simulink model "create_desRN_Test"  (R2024b)
settings: Solver=VariableStepAuto  StartTime=0.0  StopTime=10.0  RelTol=1e-3
settings Model: Creator=AdamY  LastModifiedBy=AdamY

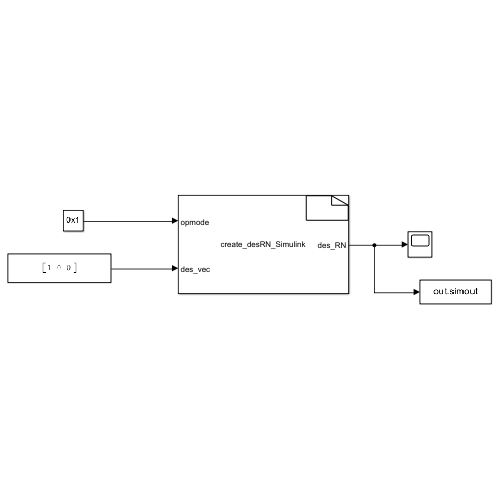
[thumbnail: Simulink's stored preview of the top-level diagram]
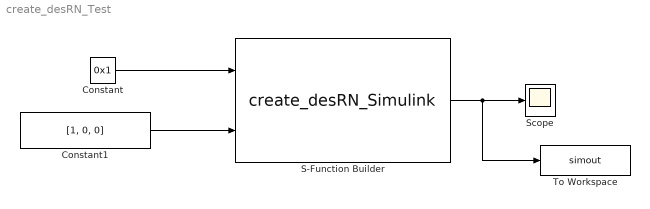
== system create_desRN_Test ==
  Constant : Constant  Value=0x1  OutDataTypeStr=uint8
  Constant1 : Constant  Value=[1, 0, 0]  OutDataTypeStr=single
  S-Function Builder : S-Function  FunctionName=create_desRN_Simulink  SFunctionModules=create_desRN_Simulink_wrapper.c att_det mtx conversions ref_rotation simulinkCustom  SFunctionDeploymentMode=off  EnableBusSupport=off  mask(S-Function Builder){}
      mask help: Simulink:masks:SFunctionBuilder_MD
      mask init:
      | val = [[.9  0.75 0.75 1 1 .9 .9 1]',[1 1 0.75 0.75 .9 .9 1 .9]'];try , sys = get_param(gcb,'SfunBuilderFcnName');if isempty(sys), sys = get_param(gcb,'FunctionName'); end,catch, sys = get_param(gcb,'FunctionName'); end
      settings: CopyFcn=set_param(gcbh,'LinkStatus','none')  OpenFcn=sfunctionwizard(gcbh)
      mask Display:
      | plot(val(:,1),val(:,2))
      | disp(sys)
      | port_label('input',1,sprintf('%s', 'opmode'),'interpreter','tex')
      | port_label('input',2,sprintf('%s', 'des\_vec'),'interpreter','tex')
      | port_label('output',1,sprintf('%s', 'des\_RN'),'interpreter','tex')
  Scope : Scope
  To Workspace : ToWorkspace  VariableName=simout  SaveFormat=Timeseries  SampleTime=-1
  wires:
  Constant/1 -> S-Function Builder/1
  S-Function Builder/1 -> To Workspace/1, Scope/1
  Constant1/1 -> S-Function Builder/2
